simulink model "Two_Wheeled_Robot_With_Default_Head_5"  (R2017b)
settings: Solver=VariableStepAuto  StartTime=0.0  StopTime=inf  RelTol=1e-3
undefined symbols (not defined in the file): Angular, Linear
libraries: simulink x4, robotlib x3
settings Model: Creator=root  LastModifiedBy=sysad

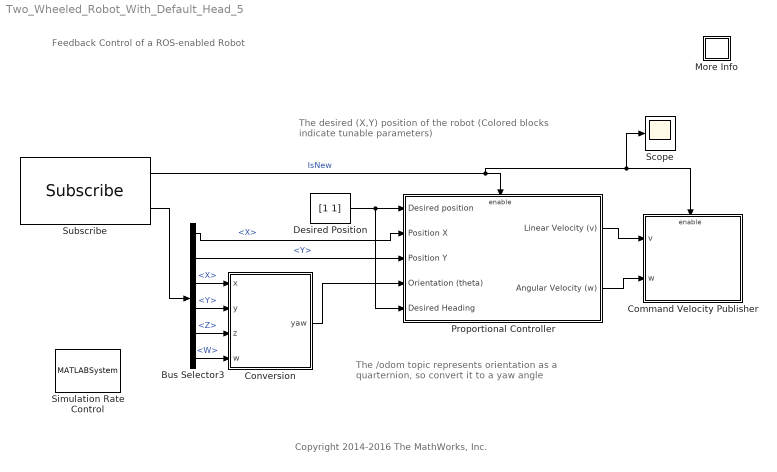
== system Two_Wheeled_Robot_With_Default_Head_5 ==
  note: Copyright 2014-2016 The MathWorks, Inc.
  note: The desired (X,Y) position of the robot
      | (Colored blocks indicate tunable parameters)
  note: The /odom topic represents orientation as a quarternion, so convert it to a yaw angle
  note: Feedback Control of a ROS-enabled Robot
  Bus Selector3 : BusSelector  OutputSignals=Pose.Pose.Position.X,Pose.Pose.Position.Y,Pose.Pose.Orientation.X,Pose.Pose.Orientation.Y,Pose.Pose.Orientation.Z,Pose.Pose.Orientation.W
  Command Velocity Publisher : Subsystem
  Conversion : MATLAB Function  TreatAsAtomicUnit=on
  Desired Position : Constant  Value=[1 1]
  More Info : Subsystem
      settings: OpenFcn=showdemo(bdroot(gcb))
      mask Display: disp('?')
  Proportional Controller : Subsystem
  Scope : Scope
  Simulation Rate Control : MATLABSystem  System=ExampleHelperSimulationRateControl  SampleTime=0.02
      mask Type: ExampleHelperSimulationRateControl
      mask Display: disp('Rate Control');
  Subscribe : robotlib/Subscribe  SourceLibraryInfo=This block requires Robotics System Toolbox  topicSource=Select from ROS network  topic=/odom  messageType=nav_msgs/Odometry  sampleTime=-1  messageQueueLength=51
      settings: SourceProductBaseCode=RO
  wires:
  Desired Position/1 -> Proportional Controller/5(Desired Heading), Proportional Controller/1(Desired position)
  Bus Selector3/2 -> Proportional Controller/3(Position Y)  "<Y>"
  Bus Selector3/4 -> Conversion/2(y)  "<Y>"
  Bus Selector3/3 -> Conversion/1(x)  "<X>"
  Subscribe/2 -> Bus Selector3/1
  Bus Selector3/6 -> Conversion/4(w)  "<W>"
  Subscribe/1 -> Command Velocity Publisher/Enable, Scope/1, Proportional Controller/Enable  "IsNew"
  Proportional Controller/1(Linear Velocity (v)) -> Command Velocity Publisher/1(v)
  Conversion/1(yaw) -> Proportional Controller/4(Orientation (theta))
  Bus Selector3/5 -> Conversion/3(z)  "<Z>"
  Proportional Controller/2(Angular Velocity (w)) -> Command Velocity Publisher/2(w)
  Bus Selector3/1 -> Proportional Controller/2(Position X)  "<X>"

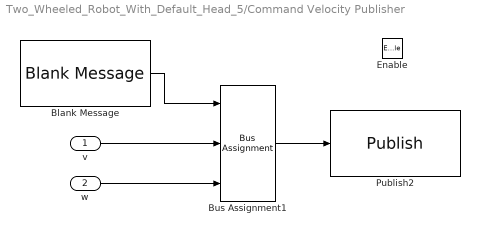
== system Two_Wheeled_Robot_With_Default_Head_5/Command Velocity Publisher ==
  v : Inport
  w : Inport  Port=2
  Enable : EnablePort
  Blank Message : robotlib/Blank Message  SourceLibraryInfo=This block requires Robotics System Toolbox  messageType=geometry_msgs/Twist  SampleTime=inf
      settings: SourceProductBaseCode=RO
  Bus Assignment1 : BusAssignment  DialogController=Simulink.DDGSource_BusAssignment  AssignedSignals=Linear.X,Angular.Z
  Publish2 : robotlib/Publish  SourceLibraryInfo=This block requires Robotics System Toolbox  topicSource=Select from ROS network  topic=/mobile_base/commands/velocity  messageType=geometry_msgs/Twist  messageQueueLength=105
      settings: SourceProductBaseCode=RO
  wires:
  Bus Assignment1/1 -> Publish2/1
  Blank Message/1 -> Bus Assignment1/1
  v/1 -> Bus Assignment1/2
  w/1 -> Bus Assignment1/3

== system Two_Wheeled_Robot_With_Default_Head_5/More Info ==

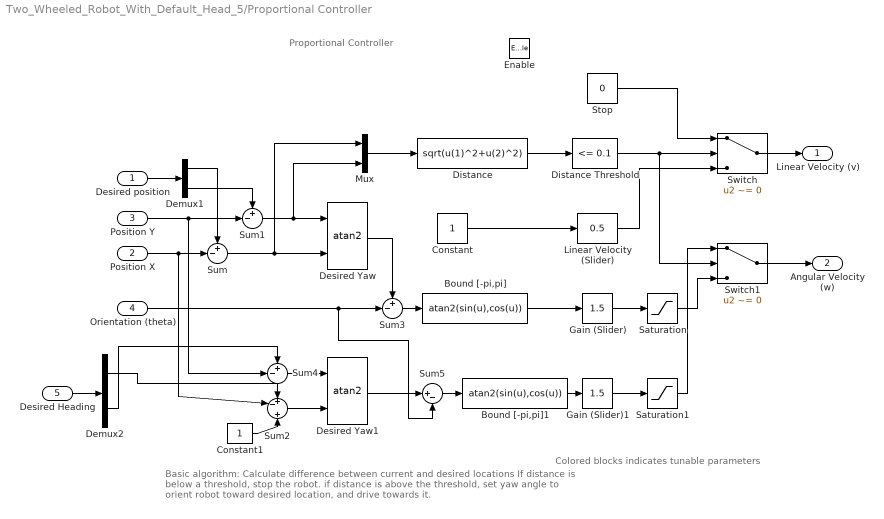
== system Two_Wheeled_Robot_With_Default_Head_5/Proportional Controller ==
  note: Proportional Controller
  note: Basic algorithm:
      | Calculate difference between current and desired locations
      | If distance is below a threshold, stop the robot.
      | if distance is above the threshold, set yaw angle to orient robot toward desired location, and drive towards it.
  note: Colored blocks indicates tunable parameters
  Desired position : Inport
  Position X : Inport  Port=2
  Position Y : Inport  Port=3
  Orientation (theta) : Inport  Port=4
  Desired Heading : Inport  Port=5
  Enable : EnablePort
  Bound [-pi,pi] : Fcn  Expr=atan2(sin(u),cos(u))
  Bound [-pi,pi]1 : Fcn  Expr=atan2(sin(u),cos(u))
  Constant : Constant
  Constant1 : Constant
  Demux1 : Demux  Outputs=2
  Demux2 : Demux  Outputs=2
  Desired Yaw : Trigonometry  Operator=atan2
  Desired Yaw1 : Trigonometry  Operator=atan2
  Distance : Fcn  Expr=sqrt(u(1)^2+u(2)^2)
  Distance Threshold : simulink/Logic and Bit Operations/Compare To Constant  relop=<=  const=0.1  OutDataTypeStr=boolean
  Gain (Slider) : simulink/Math Operations/Slider Gain  gain=1.5  low=1  high=10
  Gain (Slider)1 : simulink/Math Operations/Slider Gain  gain=1.5  low=1  high=10
  Linear Velocity (Slider) : simulink/Math Operations/Slider Gain  gain=0.5  low=0  high=2
  Mux : Mux  Inputs=2
  Saturation : Saturate
  Saturation1 : Saturate
  Stop : Constant  Value=0
  Sum{,1,3..4} (4 alike) : Sum  Inputs=+-|
  Sum2 : Sum  Inputs=+-|+
  Sum5 : Sum  Inputs=|+-
  Switch : Switch  Criteria=u2 ~= 0
  Switch1 : Switch  Criteria=u2 ~= 0
  Linear Velocity (v) : Outport
  Angular Velocity (w) : Outport  Port=2
  wires:
  Demux1/1 -> Sum/1
  Demux1/2 -> Sum1/1
  Sum1/1 -> Desired Yaw/1, Mux/2
  Desired position/1 -> Demux1/1
  Position Y/1 -> Sum4/2, Sum1/2
  Position X/1 -> Sum2/2, Sum/2
  Distance/1 -> Distance Threshold/1
  Mux/1 -> Distance/1
  Bound [-pi,pi]/1 -> Gain (Slider)/1
  Orientation (theta)/1 -> Sum5/2, Sum3/2
  Desired Yaw/1 -> Sum3/1
  Sum/1 -> Desired Yaw/2, Mux/1
  Distance Threshold/1 -> Switch1/2, Switch/2
  Gain (Slider)/1 -> Saturation/1
  Saturation/1 -> Switch1/3
  Stop/1 -> Switch/1
  Sum3/1 -> Bound [-pi,pi]/1
  Switch/1 -> Linear Velocity (v)/1
  Linear Velocity (Slider)/1 -> Switch/3
  Switch1/1 -> Angular Velocity (w)/1
  Gain (Slider)1/1 -> Saturation1/1
  Saturation1/1 -> Switch1/1
  Sum2/1 -> Desired Yaw1/2
  Sum4/1 -> Desired Yaw1/1
  Demux2/2 -> Sum4/1
  Demux2/1 -> Sum2/1
  Desired Yaw1/1 -> Sum5/1
  Sum5/1 -> Bound [-pi,pi]1/1
  Bound [-pi,pi]1/1 -> Gain (Slider)1/1
  Desired Heading/1 -> Demux2/1
  Constant/1 -> Linear Velocity (Slider)/1
  Constant1/1 -> Sum2/3

== matlab function Two_Wheeled_Robot_With_Default_Head_5/Conversion ==
  data: yaw output; x input; y input; z input; w input
function yaw  = quat2eul(x,y,z,w)
%#codegen

% Convert the quaternion to a yaw angle (zyx euler angle)
eul = quat2eul([w,x,y,z]);
yaw = eul(1);

end
